simulink model "sim_model"  (R2021b)
settings: Solver=VariableStepAuto  StartTime=0.0  StopTime=50  RelTol=1e-3
undefined symbols (not defined in the file): chi0, chi_c, g, gamma0, gamma_c, K_I_opt_new, K_P_opt_new, L_d_chi, L_d_gamma, V, w_chi, w_gamma
settings Model: Creator=hpShe  LastModifiedBy=hpShe

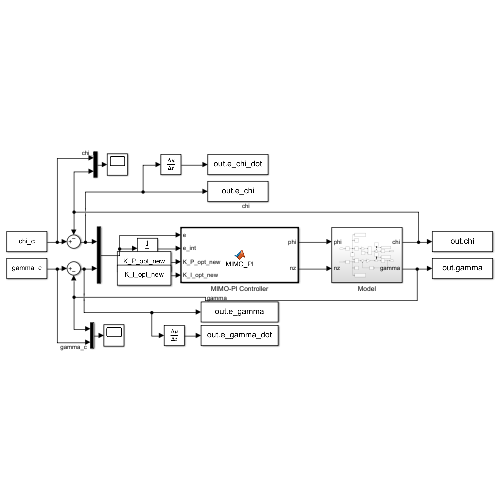
[thumbnail: Simulink's stored preview of the top-level diagram]
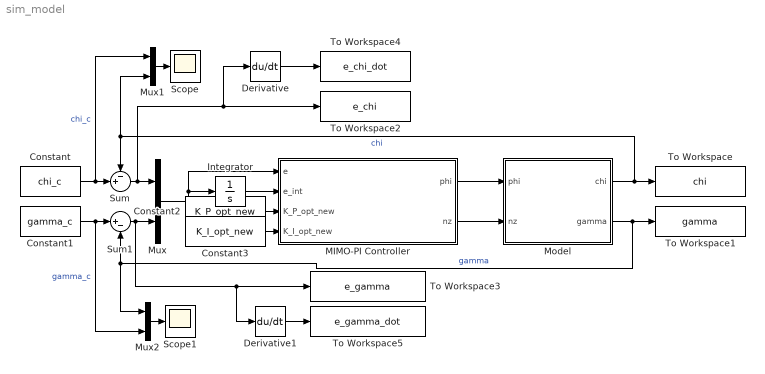
== system sim_model ==
  Constant : Constant  Value=chi_c
  Constant1 : Constant  Value=gamma_c
  Constant2 : Constant  Value=K_P_opt_new  VectorParams1D=off
  Constant3 : Constant  Value=K_I_opt_new  VectorParams1D=off
  Derivative : Derivative
  Derivative1 : Derivative
  Integrator : Integrator
  MIMO-PI Controller : MATLAB Function  TreatAsAtomicUnit=on
  Model : Subsystem
  Mux : Mux  Inputs=2
  Mux1 : Mux  Inputs=2
  Mux2 : Mux  Inputs=2
  Scope : Scope
  Scope1 : Scope
  Sum : Sum  Inputs=-+|
  Sum1 : Sum  Inputs=|+-
  To Workspace : ToWorkspace  VariableName=chi  SampleTime=-1
  To Workspace1 : ToWorkspace  VariableName=gamma  SampleTime=-1
  To Workspace2 : ToWorkspace  VariableName=e_chi  SampleTime=-1
  To Workspace3 : ToWorkspace  VariableName=e_gamma  SampleTime=-1
  To Workspace4 : ToWorkspace  VariableName=e_chi_dot  SampleTime=-1
  To Workspace5 : ToWorkspace  VariableName=e_gamma_dot  SampleTime=-1
  wires:
  Model/1(chi) -> To Workspace/1, Mux1/2, Sum/1  "chi"
  Model/2(gamma) -> Mux2/1, Sum1/2, To Workspace1/1  "gamma"
  Constant/1 -> Mux1/1, Sum/2  "chi_c"
  Constant1/1 -> Mux2/2, Sum1/1  "gamma_c"
  MIMO-PI Controller/1(phi) -> Model/1(phi)
  MIMO-PI Controller/2(nz) -> Model/2(nz)
  Sum/1 -> Derivative/1, To Workspace2/1, Mux/1
  Sum1/1 -> Derivative1/1, To Workspace3/1, Mux/2
  Mux/1 -> MIMO-PI Controller/1(e), Integrator/1
  Integrator/1 -> MIMO-PI Controller/2(e_int)
  Mux1/1 -> Scope/1
  Mux2/1 -> Scope1/1
  Constant2/1 -> MIMO-PI Controller/3(K_P_opt_new)
  Constant3/1 -> MIMO-PI Controller/4(K_I_opt_new)
  Derivative/1 -> To Workspace4/1
  Derivative1/1 -> To Workspace5/1

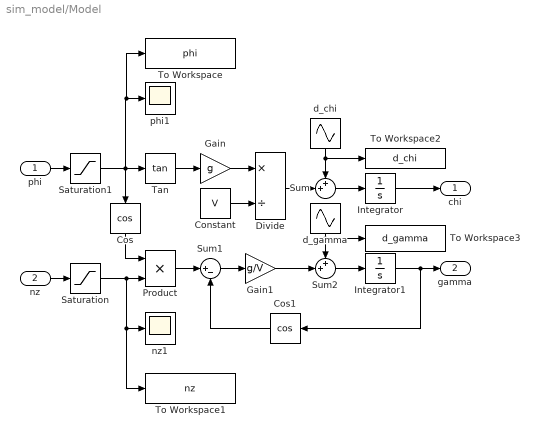
== system sim_model/Model ==
  phi : Inport
  nz : Inport  Port=2
  Constant : Constant  Value=V
  Cos : Trigonometry  Operator=cos
  Cos1 : Trigonometry  Operator=cos
  Divide : Product  Inputs=*/
  Gain : Gain  Gain=g
  Gain1 : Gain  Gain=g/V
  Integrator : Integrator  InitialCondition=chi0
  Integrator1 : Integrator  InitialCondition=gamma0
  Product : Product
  Saturation : Saturate  UpperLimit=2.1  LowerLimit=-2.1
  Saturation1 : Saturate  UpperLimit=pi/4  LowerLimit=-pi/4
  Sum : Sum  Inputs=++|
  Sum1 : Sum  Inputs=|+-
  Sum2 : Sum  Inputs=++|
  Tan : Trigonometry  Operator=tan
  To Workspace : ToWorkspace  VariableName=phi  SampleTime=-1
  To Workspace1 : ToWorkspace  VariableName=nz  SampleTime=-1
  To Workspace2 : ToWorkspace  VariableName=d_chi  SampleTime=-1
  To Workspace3 : ToWorkspace  VariableName=d_gamma  SampleTime=-1
  d_chi : Sin  Amplitude=L_d_chi  Frequency=w_chi  SampleTime=0
  d_gamma : Sin  Amplitude=L_d_gamma  Frequency=w_gamma  Phase=pi/2  SampleTime=0
  nz1 : Scope
  phi1 : Scope
  chi : Outport
  gamma : Outport  Port=2
  wires:
  Tan/1 -> Gain/1
  Gain/1 -> Divide/1
  Constant/1 -> Divide/2
  Divide/1 -> Sum/2
  d_chi/1 -> To Workspace2/1, Sum/1
  Sum/1 -> Integrator/1
  Integrator/1 -> chi/1
  Cos/1 -> Product/1
  Product/1 -> Sum1/1
  Sum1/1 -> Gain1/1
  Gain1/1 -> Sum2/2
  d_gamma/1 -> Sum2/1, To Workspace3/1
  Sum2/1 -> Integrator1/1
  Integrator1/1 -> Cos1/1, gamma/1
  Cos1/1 -> Sum1/2
  nz/1 -> Saturation/1
  Saturation/1 -> To Workspace1/1, nz1/1, Product/2
  Saturation1/1 -> To Workspace/1, phi1/1, Cos/1, Tan/1
  phi/1 -> Saturation1/1

== matlab function sim_model/MIMO-PI Controller ==
  data: e input; e_int input; phi output; nz output; K_P_opt_new input; K_I_opt_new input
function [phi,nz] = MIMO_PI(e,e_int,K_P_opt_new,K_I_opt_new)
    u = K_P_opt_new * e + K_I_opt_new * e_int;
%     disp('---------------------------------');
%     disp(['e:']); disp(e);
%     disp(['e_integral:']); disp(e_int);
%     disp(['K_P_opt_new:']); disp(K_P_opt_new);
%     disp(['K_I_opt_new:']); disp(K_I_opt_new);
     phi = u(1); 
     nz = u(2);
end
